simulink model "Bibelmodel"  (R2022a)
settings: Solver=VariableStepAuto  StartTime=0.0  StopTime=simtime  RelTol=1e-3
values from neighbouring files (symbols this model uses):
  A_Veh = 1.05    [params.m]
  coeff_DragLoad_Frnt = 0.1    [params.m]
  coeff_DragLoad_Re = 0.1    [params.m]
  coeff_LiftLoad_Frnt = 0.53    [params.m]
  coeff_LiftLoad_Re = 0.53    [params.m]
  coeff_Veh_Drag = 1.35    [params.m]
  coeff_Veh_Lift = 5.2    [params.m]
  coeff_WhlLoad_Frnt = 0.466    [params.m]
  coeff_WhlLoad_Re = 0.534    [params.m]
  dens_Air = 1.2041    [params.m]
  diam_Pist_Frnt = 2.54    [params.m]
  diam_Pist_Re = 2.54    [params.m]
  dst_Track_Frnt = 0.5    [params.m]
  dst_Track_Re = 0.5    [params.m]
  dst_WhlBase_Frnt = 0.714    [params.m]
  dst_WhlBase_Re = 0.821    [params.m]
  height_Cog = 0.25    [params.m]
  I_Mot = 1    [params.m]
  I_Veh = 80    [params.m]
  I_Whl = 2    [params.m]
  initial_speed = max(v_acc) / 3.6    [laptimeV1.m]
  m_Veh = 290    [params.m]
  mu_Brk = 0.56    [params.m]
  nu_Pist_Frnt = 4    [params.m]
  nu_Pist_Re = 2    [params.m]
  rad_BrkDisc_Frnt = 0.1725    [params.m]
  rad_BrkDisc_Re = 0.1725    [params.m]
  rad_Tire_Dyn = 0.2032    [params.m]
  rat_Gbx = 13.8    [params.m]
undefined symbols (not defined in the file or in its folder): initial_yaw
settings Model: SimulationMode=accelerator  Creator=gbour  LastModifiedBy=gbour
settings DebuggingCC: UnderSpecifiedDimensionMsg=warning

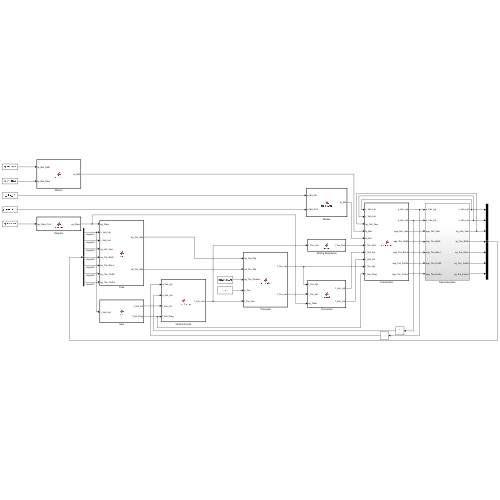
[thumbnail: Simulink's stored preview of the top-level diagram]
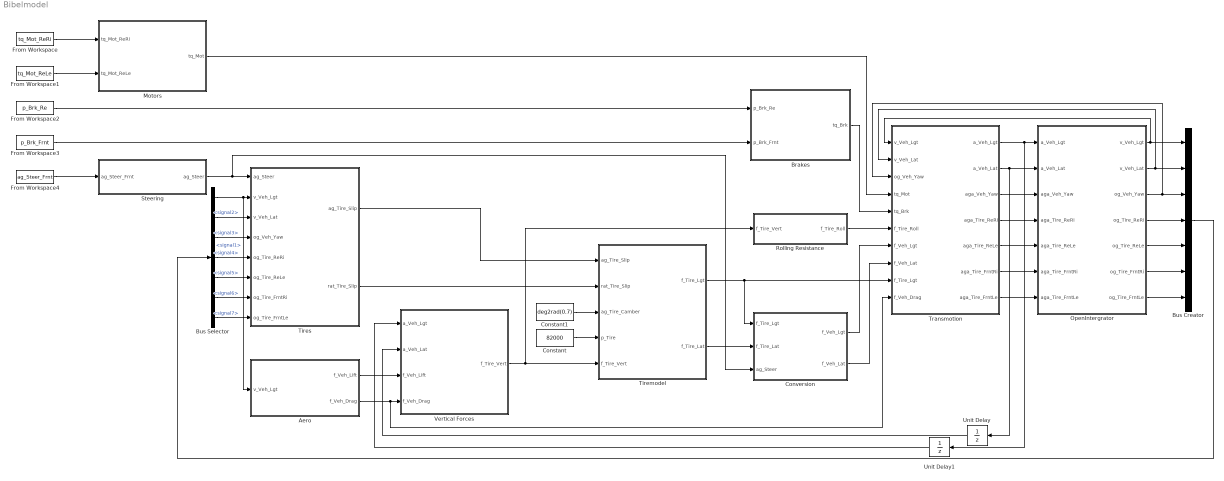
== system Bibelmodel ==
  Aero : MATLAB Function  TreatAsAtomicUnit=on
  Brakes : MATLAB Function  TreatAsAtomicUnit=on
  Bus Creator : BusCreator  Inputs=7
  Bus Selector : BusSelector  OutputSignals=signal1,signal2,signal3,signal4,signal5,signal6,signal7
  Constant : Constant  Value=82000
  Constant1 : Constant  Value=deg2rad(0.7)
  Conversion : MATLAB Function  TreatAsAtomicUnit=on
  From Workspace : FromWorkspace  VariableName=tq_Mot_ReRi
  From Workspace1 : FromWorkspace  VariableName=tq_Mot_ReLe
  From Workspace2 : FromWorkspace  VariableName=p_Brk_Re
  From Workspace3 : FromWorkspace  VariableName=p_Brk_Frnt
  From Workspace4 : FromWorkspace  VariableName=ag_Steer_Frnt
  Motors : MATLAB Function  TreatAsAtomicUnit=on
  OpenIntergrator : Subsystem
  Rolling Resistance : MATLAB Function  TreatAsAtomicUnit=on
  Steering : MATLAB Function  TreatAsAtomicUnit=on
  Tiremodel : MATLAB Function  TreatAsAtomicUnit=on
  Tires : MATLAB Function  TreatAsAtomicUnit=on
  Transmotion : MATLAB Function  TreatAsAtomicUnit=on
  Unit Delay : UnitDelay  SampleTime=-1  HasFrameUpgradeWarning=on
  Unit Delay1 : UnitDelay  SampleTime=-1  HasFrameUpgradeWarning=on
  Vertical Forces : MATLAB Function  TreatAsAtomicUnit=on
  wires:
  Transmotion/1(a_Veh_Lgt) -> Unit Delay1/1, OpenIntergrator/1(a_Veh_Lgt)
  Transmotion/2(a_Veh_Lat) -> Unit Delay/1, OpenIntergrator/2(a_Veh_Lat)
  Transmotion/3(aga_Veh_Yaw) -> OpenIntergrator/3(aga_Veh_Yaw)
  Transmotion/4(aga_Tire_ReRi) -> OpenIntergrator/4(aga_Tire_ReRi)
  Transmotion/5(aga_Tire_ReLe) -> OpenIntergrator/5(aga_Tire_ReLe)
  Transmotion/6(aga_Tire_FrntRi) -> OpenIntergrator/6(aga_Tire_FrntRi)
  Transmotion/7(aga_Tire_FrntLe) -> OpenIntergrator/7(aga_Tire_FrntLe)
  Tiremodel/1(f_Tire_Lgt) -> Conversion/1(f_Tire_Lgt), Transmotion/9(f_Tire_Lgt)
  Vertical Forces/1(f_Tire_Vert) -> Rolling Resistance/1(f_Tire_Vert), Tiremodel/5(f_Tire_Vert)
  Aero/1(f_Veh_Lift) -> Vertical Forces/3(f_Veh_Lift)
  Aero/2(f_Veh_Drag) -> Transmotion/10(f_Veh_Drag), Vertical Forces/4(f_Veh_Drag)
  OpenIntergrator/1(v_Veh_Lgt) -> Transmotion/1(v_Veh_Lgt), Bus Creator/1
  OpenIntergrator/2(v_Veh_Lat) -> Bus Creator/2, Transmotion/2(v_Veh_Lat)
  OpenIntergrator/3(og_Veh_Yaw) -> Transmotion/3(og_Veh_Yaw), Bus Creator/3
  Constant/1 -> Tiremodel/4(p_Tire)
  Constant1/1 -> Tiremodel/3(ag_Tire_Camber)
  Steering/1(ag_Steer) -> Conversion/3(ag_Steer), Tires/1(ag_Steer)
  Tires/1(ag_Tire_Slip) -> Tiremodel/1(ag_Tire_Slip)
  Tires/2(rat_Tire_Slip) -> Tiremodel/2(rat_Tire_Slip)
  OpenIntergrator/7(og_Tire_FrntLe) -> Bus Creator/7
  OpenIntergrator/6(og_Tire_FrntRi) -> Bus Creator/6
  OpenIntergrator/5(og_Tire_ReLe) -> Bus Creator/5
  OpenIntergrator/4(og_Tire_ReRi) -> Bus Creator/4
  Bus Creator/1 -> Bus Selector/1
  Bus Selector/7 -> Tires/8(og_Tire_FrntLe)  "<signal7>"
  Bus Selector/6 -> Tires/7(og_Tire_FrntRi)  "<signal6>"
  Bus Selector/5 -> Tires/6(og_Tire_ReLe)  "<signal5>"
  Bus Selector/4 -> Tires/5(og_Tire_ReRi)  "<signal4>"
  Bus Selector/3 -> Tires/4(og_Veh_Yaw)  "<signal3>"
  Bus Selector/2 -> Tires/3(v_Veh_Lat)  "<signal2>"
  Bus Selector/1 -> Aero/1(v_Veh_Lgt), Tires/2(v_Veh_Lgt)  "<signal1>"
  Tiremodel/2(f_Tire_Lat) -> Conversion/2(f_Tire_Lat)
  Conversion/1(f_Veh_Lgt) -> Transmotion/7(f_Veh_Lgt)
  Conversion/2(f_Veh_Lat) -> Transmotion/8(f_Veh_Lat)
  Rolling Resistance/1(f_Tire_Roll) -> Transmotion/6(f_Tire_Roll)
  Unit Delay/1 -> Vertical Forces/2(a_Veh_Lat)
  Unit Delay1/1 -> Vertical Forces/1(a_Veh_Lgt)
  Brakes/1(tq_Brk) -> Transmotion/5(tq_Brk)
  From Workspace4/1 -> Steering/1(ag_Steer_Frnt)
  From Workspace3/1 -> Brakes/2(p_Brk_Frnt)
  From Workspace2/1 -> Brakes/1(p_Brk_Re)
  From Workspace1/1 -> Motors/2(tq_Mot_ReLe)
  From Workspace/1 -> Motors/1(tq_Mot_ReRi)
  Motors/1(tq_Mot) -> Transmotion/4(tq_Mot)

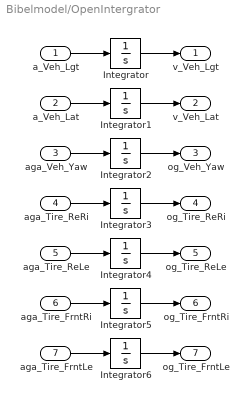
== system Bibelmodel/OpenIntergrator ==
  a_Veh_Lgt : Inport
  a_Veh_Lat : Inport  Port=2
  aga_Veh_Yaw : Inport  Port=3
  aga_Tire_ReRi : Inport  Port=4
  aga_Tire_ReLe : Inport  Port=5
  aga_Tire_FrntRi : Inport  Port=6
  aga_Tire_FrntLe : Inport  Port=7
  Integrator : Integrator  InitialCondition=initial_speed
  Integrator1 : Integrator
  Integrator2 : Integrator  InitialCondition=initial_yaw
  Integrator{3..6} (4 alike) : Integrator  InitialCondition=initial_speed / rad_Tire_Dyn
  v_Veh_Lgt : Outport
  v_Veh_Lat : Outport  Port=2
  og_Veh_Yaw : Outport  Port=3
  og_Tire_ReRi : Outport  Port=4
  og_Tire_ReLe : Outport  Port=5
  og_Tire_FrntRi : Outport  Port=6
  og_Tire_FrntLe : Outport  Port=7
  wires:
  Integrator6/1 -> og_Tire_FrntLe/1
  Integrator4/1 -> og_Tire_ReLe/1
  Integrator/1 -> v_Veh_Lgt/1
  Integrator2/1 -> og_Veh_Yaw/1
  aga_Tire_ReLe/1 -> Integrator4/1
  aga_Tire_FrntRi/1 -> Integrator5/1
  Integrator3/1 -> og_Tire_ReRi/1
  Integrator5/1 -> og_Tire_FrntRi/1
  a_Veh_Lat/1 -> Integrator1/1
  aga_Veh_Yaw/1 -> Integrator2/1
  aga_Tire_ReRi/1 -> Integrator3/1
  aga_Tire_FrntLe/1 -> Integrator6/1
  a_Veh_Lgt/1 -> Integrator/1
  Integrator1/1 -> v_Veh_Lat/1

== matlab function Bibelmodel/Steering ==
  data: ag_Steer_Frnt input size=1; ag_Steer output size=[4 1]
function ag_Steer = steering(ag_Steer_Frnt)

ag_Steer = zeros(4, 1);

ag_Steer(3) = ag_Steer_Frnt;
ag_Steer(4) = ag_Steer_Frnt;

end

== matlab function Bibelmodel/Tires ==
  data: ag_Steer input size=[4 1]; v_Veh_Lgt input size=1; ag_Tire_Slip output size=[4 1]; rat_Tire_Slip output size=[4 1]; v_Veh_Lat input size=1; og_Veh_Yaw input size=1; og_Tire_ReRi input size=1; og_Tire_ReLe input size=1; og_Tire_FrntRi input size=1; og_Tire_FrntLe input size=1; rad_Tire_Dyn parameter size=1; dst_Track_Re parameter size=1; dst_Track_Frnt parameter size=1; dst_WhlBase_Re parameter size=1; dst_WhlBase_Frnt parameter size=1
function [ag_Tire_Slip, rat_Tire_Slip] = tires(ag_Steer, v_Veh_Lgt, v_Veh_Lat, og_Veh_Yaw, og_Tire_ReRi, og_Tire_ReLe, og_Tire_FrntRi, og_Tire_FrntLe, rad_Tire_Dyn, dst_Track_Re, dst_Track_Frnt, dst_WhlBase_Re, dst_WhlBase_Frnt)

temp_Lgt = v_Veh_Lgt + (og_Veh_Yaw .* [dst_Track_Re; -dst_Track_Re; dst_Track_Frnt; -dst_Track_Frnt]);
temp_Lat = v_Veh_Lat + (og_Veh_Yaw .* [dst_WhlBase_Re; -dst_WhlBase_Re; dst_WhlBase_Frnt; -dst_WhlBase_Frnt]);

v_Tire_Lgt = (temp_Lgt .* cos(ag_Steer)) + (temp_Lat .* sin(ag_Steer));
v_Tire_Lat = (-temp_Lgt .* sin(ag_Steer)) + (temp_Lat .* cos(ag_Steer));

og_Tire = [og_Tire_ReRi; og_Tire_ReLe; og_Tire_FrntRi; og_Tire_FrntLe];

ag_Tire_Slip = atan(v_Tire_Lat ./ v_Tire_Lgt);
rat_Tire_Slip = ((og_Tire .* rad_Tire_Dyn) - v_Tire_Lgt) ./ v_Tire_Lgt;

end

== matlab function Bibelmodel/Conversion ==
  data: f_Tire_Lgt input size=[4 1]; f_Veh_Lgt output size=[4 1]; f_Tire_Lat input size=[4 1]; ag_Steer input size=[4 1]; f_Veh_Lat output size=[4 1]
function [f_Veh_Lgt, f_Veh_Lat] = conversion(f_Tire_Lgt, f_Tire_Lat, ag_Steer)

f_Veh_Lgt = f_Tire_Lgt .* cos(ag_Steer) - f_Tire_Lat .* sin(ag_Steer);
f_Veh_Lat = f_Tire_Lgt .* sin(ag_Steer) + f_Tire_Lat .* cos(ag_Steer);

end

== matlab function Bibelmodel/Rolling Resistance ==
  data: f_Tire_Vert input size=[4 1]; f_Tire_Roll output size=[4 1]; coeff_Roll parameter size=1
function f_Tire_Roll = rollres(f_Tire_Vert, coeff_Roll)

f_Tire_Roll = f_Tire_Vert * coeff_Roll;

end

== matlab function Bibelmodel/Brakes ==
  data: p_Brk_Re input size=1; tq_Brk output size=[4 1]; p_Brk_Frnt input size=1; diam_Pist_Re parameter size=1; diam_Pist_Frnt parameter size=1; nu_Pist_Re parameter size=1; nu_Pist_Frnt parameter size=1; rad_BrkDisc_Re parameter size=1; rad_BrkDisc_Frnt parameter size=1; mu_Brk parameter size=1
function tq_Brk = rearbrakes(p_Brk_Re, p_Brk_Frnt, diam_Pist_Re, diam_Pist_Frnt, nu_Pist_Re, nu_Pist_Frnt, rad_BrkDisc_Re, rad_BrkDisc_Frnt, mu_Brk)

tq_Brk = zeros(4, 1);

tq_Brk(1) = - 0.5 * (((pi * p_Brk_Re * ((diam_Pist_Re^2) / 4)) * nu_Pist_Re * mu_Brk) * 0.5 * rad_BrkDisc_Re);
tq_Brk(2) = - 0.5 * (((pi * p_Brk_Re * ((diam_Pist_Re^2) / 4)) * nu_Pist_Re * mu_Brk) * 0.5 * rad_BrkDisc_Re);
tq_Brk(3) = - 0.5 * (((pi * p_Brk_Frnt * ((diam_Pist_Frnt^2) / 4)) * nu_Pist_Frnt * mu_Brk) * 0.5 * rad_BrkDisc_Frnt);
tq_Brk(4) = - 0.5 * (((pi * p_Brk_Frnt * ((diam_Pist_Frnt^2) / 4)) * nu_Pist_Frnt * mu_Brk) * 0.5 * rad_BrkDisc_Frnt);

end

== matlab function Bibelmodel/Motors ==
  data: tq_Mot_ReRi input size=1; tq_Mot output size=[2 1]; tq_Mot_ReLe input size=1
function tq_Mot = motors(tq_Mot_ReRi, tq_Mot_ReLe)

tq_Mot = zeros(2, 1);

tq_Mot(1) = tq_Mot_ReRi;
tq_Mot(2) = tq_Mot_ReLe;

end

== matlab function Bibelmodel/Tiremodel ==
  data: ag_Tire_Slip input size=[4 1]; f_Tire_Lgt output size=[4 1]; rat_Tire_Slip input size=[4 1]; ag_Tire_Camber input size=1; p_Tire input size=1; f_Tire_Vert input size=[4 1]; f_Tire_Lat output size=[4 1]
function [f_Tire_Lgt, f_Tire_Lat] = tiremodel(ag_Tire_Slip, rat_Tire_Slip, ag_Tire_Camber, p_Tire, f_Tire_Vert)

coder.extrinsic('magicformula.v62.eval')

f_Tire_Lgt = zeros(4, 1);
f_Tire_Lat = zeros(4, 1);

[f_Tire_Lgt(1), f_Tire_Lat(1), ~, ~] = magicformula.v62.eval(ag_Tire_Slip(1), rat_Tire_Slip(1), ag_Tire_Camber, p_Tire, f_Tire_Vert(1), 1);
[f_Tire_Lgt(2), f_Tire_Lat(2), ~, ~] = magicformula.v62.eval(ag_Tire_Slip(2), rat_Tire_Slip(2), ag_Tire_Camber, p_Tire, f_Tire_Vert(2), 0);
[f_Tire_Lgt(3), f_Tire_Lat(3), ~, ~] = magicformula.v62.eval(ag_Tire_Slip(3), rat_Tire_Slip(3), ag_Tire_Camber, p_Tire, f_Tire_Vert(3), 1);
[f_Tire_Lgt(4), f_Tire_Lat(4), ~, ~] = magicformula.v62.eval(ag_Tire_Slip(4), rat_Tire_Slip(4), ag_Tire_Camber, p_Tire, f_Tire_Vert(4), 0);

end

== matlab function Bibelmodel/Transmotion ==
  data: v_Veh_Lgt input size=1; v_Veh_Lat input size=1; og_Veh_Yaw input size=1; tq_Mot input size=[2 1]; tq_Brk input size=[4 1]; f_Tire_Roll input size=[4 1]; f_Veh_Lgt input size=[4 1]; a_Veh_Lgt output size=1; a_Veh_Lat output size=1; aga_Veh_Yaw output size=1; aga_Tire_ReRi output size=1; aga_Tire_ReLe output size=1; aga_Tire_FrntRi output size=1; aga_Tire_FrntLe output size=1; f_Veh_Lat input size=[4 1]; f_Tire_Lgt input size=[4 1]; f_Veh_Drag input size=1; m_Veh parameter size=1; I_Veh parameter size=1; dst_Track_Frnt parameter size=1; dst_Track_Re parameter size=1; dst_WhlBase_Frnt parameter size=1; dst_WhlBase_Re parameter size=1; rat_Gbx parameter size=1; rad_Tire_Dyn parameter size=1; I_Whl parameter size=1; I_Mot parameter size=1
function [a_Veh_Lgt, a_Veh_Lat, aga_Veh_Yaw, aga_Tire_ReRi, aga_Tire_ReLe, aga_Tire_FrntRi, aga_Tire_FrntLe] = transmotion(v_Veh_Lgt, v_Veh_Lat, og_Veh_Yaw, tq_Mot, tq_Brk, f_Tire_Roll, f_Veh_Lgt, f_Veh_Lat, f_Tire_Lgt, f_Veh_Drag, m_Veh, I_Veh, dst_Track_Frnt, dst_Track_Re, dst_WhlBase_Frnt, dst_WhlBase_Re, rat_Gbx, rad_Tire_Dyn, I_Whl, I_Mot)

a_Veh_Lgt = (1 / m_Veh) * sum(f_Veh_Lgt - f_Veh_Drag) + og_Veh_Yaw * v_Veh_Lat;
a_Veh_Lat = (1 / m_Veh) * sum(f_Veh_Lat) - og_Veh_Yaw * v_Veh_Lgt;

aga_Veh_Yaw = (1 / I_Veh) * (0.5 * dst_Track_Frnt * (f_Veh_Lgt(2) - f_Veh_Lgt(1) + 0.5 * dst_Track_Re * (f_Veh_Lgt(4) - f_Veh_Lgt(3))) ...
    + dst_WhlBase_Frnt * (f_Veh_Lat(1) + f_Veh_Lat(2)) - dst_WhlBase_Re * (f_Veh_Lat(3) + f_Veh_Lat(4)));

aga_Tire_ReRi = (rat_Gbx * tq_Mot(1) + tq_Brk(1) - (f_Tire_Lgt(1) - f_Tire_Roll(1)) * rad_Tire_Dyn) / (I_Whl + rat_Gbx^2 * I_Mot);
aga_Tire_ReLe = (rat_Gbx * tq_Mot(2) + tq_Brk(2) - (f_Tire_Lgt(2) - f_Tire_Roll(2)) * rad_Tire_Dyn) / (I_Whl + rat_Gbx^2 * I_Mot);
aga_Tire_FrntRi = (tq_Brk(3) - (f_Tire_Lgt(3) - f_Tire_Roll(3)) * rad_Tire_Dyn) / (I_Whl);
aga_Tire_FrntLe = (tq_Brk(4) - (f_Tire_Lgt(4) - f_Tire_Roll(4)) * rad_Tire_Dyn) / (I_Whl);

end

== matlab function Bibelmodel/Aero ==
  data: v_Veh_Lgt input size=1; f_Veh_Lift output size=1; f_Veh_Drag output size=1; dens_Air parameter size=1; A_Veh parameter size=1; coeff_Veh_Lift parameter size=1; coeff_Veh_Drag parameter size=1
function [f_Veh_Lift, f_Veh_Drag] = aero(v_Veh_Lgt, dens_Air, A_Veh, coeff_Veh_Lift, coeff_Veh_Drag)

f_Veh_Lift = 0.5 * dens_Air * A_Veh * coeff_Veh_Lift * v_Veh_Lgt^2;
f_Veh_Drag = 0.5 * dens_Air * A_Veh * coeff_Veh_Drag * v_Veh_Lgt^2;

end

== matlab function Bibelmodel/Vertical Forces ==
  data: a_Veh_Lgt input size=1; f_Tire_Vert output size=[4 1]; a_Veh_Lat input size=1; f_Veh_Lift input size=1; f_Veh_Drag input size=1; coeff_WhlLoad_Re parameter size=1; coeff_WhlLoad_Frnt parameter size=1; m_Veh parameter size=1; height_Cog parameter size=1; dst_Track_Re parameter size=1; dst_Track_Frnt parameter size=1; dst_WhlBase_Re parameter size=1; dst_WhlBase_Frnt parameter size=1; coeff_LiftLoad_Re parameter size=1; coeff_LiftLoad_Frnt parameter size=1; coeff_DragLoad_Re parameter size=1; coeff_DragLoad_Frnt parameter size=1
function f_Tire_Vert = verticalforces(a_Veh_Lgt, a_Veh_Lat, f_Veh_Lift, f_Veh_Drag, coeff_WhlLoad_Re, coeff_WhlLoad_Frnt, m_Veh, height_Cog, dst_Track_Re, dst_Track_Frnt, dst_WhlBase_Re, dst_WhlBase_Frnt, coeff_LiftLoad_Re, coeff_LiftLoad_Frnt, coeff_DragLoad_Re, coeff_DragLoad_Frnt)

f_Tire_Vert = zeros(4, 1);

f_Tire_Vert(1) = (0.5 * m_Veh * 9.81 * coeff_WhlLoad_Re) + (0.5 * m_Veh * coeff_WhlLoad_Re * a_Veh_Lat * height_Cog / dst_Track_Re) ...
    + (0.5 * m_Veh * coeff_WhlLoad_Re * a_Veh_Lgt * height_Cog / dst_WhlBase_Re) + (0.5 * f_Veh_Lift * coeff_LiftLoad_Re) + (0.5 * f_Veh_Drag * coeff_DragLoad_Re);

f_Tire_Vert(2) = (0.5 * m_Veh * 9.81 * coeff_WhlLoad_Re) - (0.5 * m_Veh * coeff_WhlLoad_Re * a_Veh_Lat * height_Cog / dst_Track_Re) ...
    - (0.5 * m_Veh * coeff_WhlLoad_Re * a_Veh_Lgt * height_Cog / dst_WhlBase_Re) + (0.5 * f_Veh_Lift * coeff_LiftLoad_Re) + (0.5 * f_Veh_Drag * coeff_DragLoad_Re);

f_Tire_Vert(3) = (0.5 * m_Veh * 9.81 * coeff_WhlLoad_Frnt) + (0.5 * m_Veh * coeff_WhlLoad_Frnt * a_Veh_Lat * height_Cog / dst_Track_Frnt) ...
    + (0.5 * m_Veh * coeff_WhlLoad_Frnt * a_Veh_Lgt * height_Cog / dst_WhlBase_Frnt) + (0.5 * f_Veh_Lift * coeff_LiftLoad_Frnt) - (0.5 * f_Veh_Drag * coeff_DragLoad_Frnt);

f_Tire_Vert(4) = (0.5 * m_Veh * 9.81 * coeff_WhlLoad_Frnt) - (0.5 * m_Veh * coeff_WhlLoad_Frnt * a_Veh_Lat * height_Cog / dst_Track_Frnt) ...
    - (0.5 * m_Veh * coeff_WhlLoad_Frnt * a_Veh_Lgt * height_Cog / dst_WhlBase_Frnt) + (0.5 * f_Veh_Lift * coeff_LiftLoad_Frnt) - (0.5 * f_Veh_Drag * coeff_DragLoad_Frnt);

end
